simulink model "branch_offset_rate210_20161217_000202"  (R2014a)
settings: Solver=FixedStepDiscrete  SolverMode=SingleTasking  StartTime=0.0  StopTime=10.0  FixedStep=0.002  RelTol=1e-3
settings Model: BufferReuse=off  Creator=yoshi12  LastModifiedBy=yoshi12
settings OptimizationCC: BlockReduction=off  OptimizeBlockIOStorage=off  BufferReuse=off  GlobalBufferReuse=off  ExpressionFolding=off  LocalBlockOutputs=off  OptimizeModelRefInitCode=on  LifeSpan=1  SimCompilerOptimization=off
settings DebuggingCC: MergeDetectMultiDrivingBlocksExec=error  MultiTaskRateTransMsg=warning  FrameProcessingCompatibilityMsg=error
settings RTWCC: SystemTargetFile=ert.tlc  GenCodeOnly=on  TemplateMakefile=ert_default_tmf  Description=Embedded Coder  GenerateReport=on  IncludeHyperlinkInReport=on  LaunchReport=on  GenerateTraceInfo=on  GenerateTraceReport=on  GenerateTraceReportSl=on  GenerateTraceReportSf=on  GenerateTraceReportEml=on  RTWCompilerOptimization=off
settings CodeAppCC: IgnoreCustomStorageClasses=off
settings ERTTargetCC: ParMdlRefBuildCompliant=on  CompOptLevelCompliant=on  ConcurrentExecutionCompliant=on  ERTFirstTimeCompliant=on  ModelStepFunctionPrototypeControlCompliant=on  CPPClassGenCompliant=on  InlinedParameterPlacement=Hierarchical  ERTCustomFileTemplate=example_file_process.tlc
settings ConfigComp: CovMetricSettings=dw  CovHtmlReporting=on  CovSaveCumulativeToWorkspaceVar=on  CovSaveSingleToWorkspaceVar=on  CovModelRefEnable=Off  CovExternalEMLEnable=off  CovSFcnEnable=off

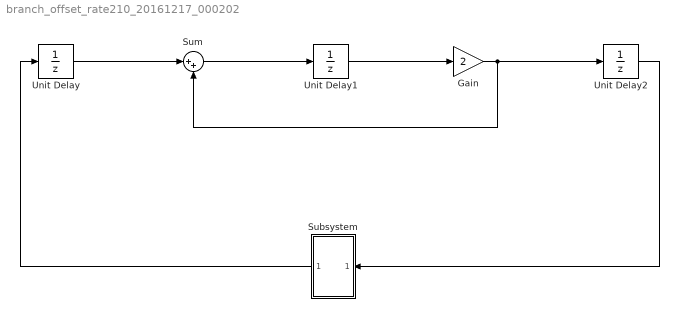
== system branch_offset_rate210_20161217_000202 ==
  Gain : Gain  Gain=2  SampleTime=0.002
  Subsystem : Subsystem
  Sum : Sum  Inputs=|++  SampleTime=0.002
  Unit Delay : UnitDelay  InitialCondition=1  SampleTime=-1
  Unit Delay1 : UnitDelay  InitialCondition=2  SampleTime=-1
  Unit Delay2 : UnitDelay  InitialCondition=1  SampleTime=-1
  wires:
  Unit Delay/1 -> Sum/1
  Sum/1 -> Unit Delay1/1
  Unit Delay1/1 -> Gain/1
  Gain/1 -> Sum/2, Unit Delay2/1
  Unit Delay2/1 -> Subsystem/1(In1)
  Subsystem/1(Out1) -> Unit Delay/1

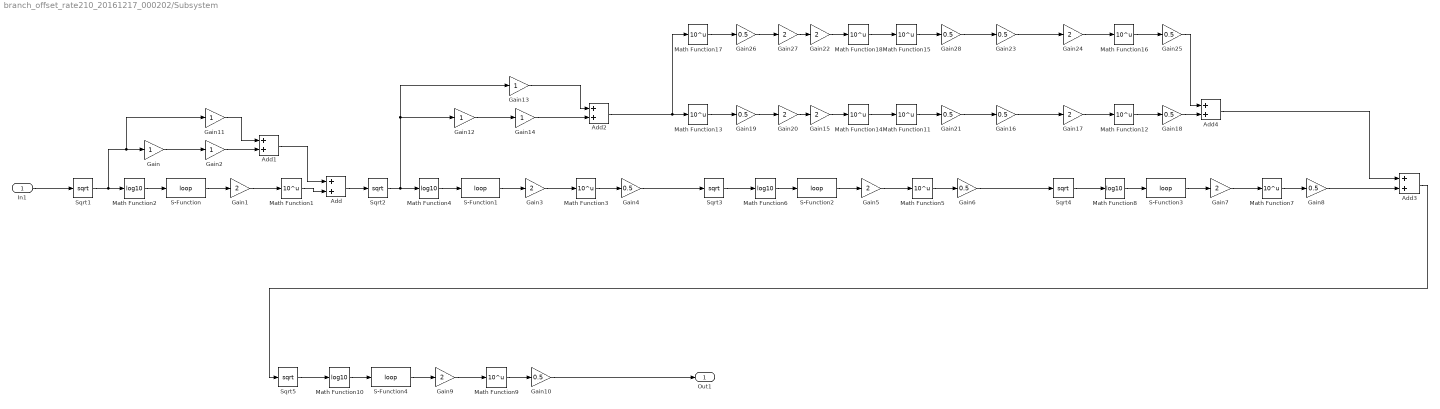
== system branch_offset_rate210_20161217_000202/Subsystem ==
  In1 : Inport
  Add{,1..2,4} (4 alike) : Sum  SampleTime=[0.01,0]
  Add3 : Sum  SampleTime=[0.01,0.006]
  Gain{,2,11..14} (6 alike) : Gain  SampleTime=[0.01,0]
  Gain1 : Gain  Gain=2  SampleTime=[0.01,0]
  Gain10 : Gain  Gain=0.5  SampleTime=[0.01,0.008]
  Gain{7,15,17,20,22,24,27} (7 alike) : Gain  Gain=2  SampleTime=[0.01,0.006]
  Gain{8,16,18..19,21,23,25..26,28} (9 alike) : Gain  Gain=0.5  SampleTime=[0.01,0.006]
  Gain3 : Gain  Gain=2  SampleTime=[0.01,0.002]
  Gain4 : Gain  Gain=0.5  SampleTime=[0.01,0.002]
  Gain5 : Gain  Gain=2  SampleTime=[0.01,0.004]
  Gain6 : Gain  Gain=0.5  SampleTime=[0.01,0.004]
  Gain9 : Gain  Gain=2  SampleTime=[0.01,0.008]
  Math Function1 : Math  Operator=10^u  SampleTime=[0.01,0]  SaturateOnIntegerOverflow=on
  Math Function10 : Math  Operator=log10  SampleTime=[0.01,0.008]  SaturateOnIntegerOverflow=on
  Math Function{7,11..18} (9 alike) : Math  Operator=10^u  SampleTime=[0.01,0.006]  SaturateOnIntegerOverflow=on
  Math Function2 : Math  Operator=log10  SampleTime=[0.01,0]  SaturateOnIntegerOverflow=on
  Math Function3 : Math  Operator=10^u  SampleTime=[0.01,0.002]  SaturateOnIntegerOverflow=on
  Math Function4 : Math  Operator=log10  SampleTime=[0.01,0.002]  SaturateOnIntegerOverflow=on
  Math Function5 : Math  Operator=10^u  SampleTime=[0.01,0.004]  SaturateOnIntegerOverflow=on
  Math Function6 : Math  Operator=log10  SampleTime=[0.01,0.004]  SaturateOnIntegerOverflow=on
  Math Function8 : Math  Operator=log10  SampleTime=[0.01,0.006]  SaturateOnIntegerOverflow=on
  Math Function9 : Math  Operator=10^u  SampleTime=[0.01,0.008]  SaturateOnIntegerOverflow=on
  S-Function{,1..4} (5 alike) : S-Function  FunctionName=loop  EnableBusSupport=off
  Sqrt1 : Sqrt  SampleTime=[0.01,0]  SaturateOnIntegerOverflow=on
  Sqrt2 : Sqrt  SampleTime=[0.01,0.002]  SaturateOnIntegerOverflow=on
  Sqrt3 : Sqrt  SampleTime=[0.01,0.004]  SaturateOnIntegerOverflow=on
  Sqrt4 : Sqrt  SampleTime=[0.01,0.006]  SaturateOnIntegerOverflow=on
  Sqrt5 : Sqrt  SampleTime=[0.01,0.008]  SaturateOnIntegerOverflow=on
  Out1 : Outport
  wires:
  Math Function3/1 -> Gain4/1
  Math Function8/1 -> S-Function3/1
  Sqrt1/1 -> Gain11/1, Gain/1, Math Function2/1
  Math Function10/1 -> S-Function4/1
  Gain9/1 -> Math Function9/1
  Math Function1/1 -> Add/2
  S-Function2/1 -> Gain5/1
  Math Function9/1 -> Gain10/1
  Gain10/1 -> Out1/1
  Sqrt3/1 -> Math Function6/1
  Sqrt4/1 -> Math Function8/1
  Gain3/1 -> Math Function3/1
  Gain6/1 -> Sqrt4/1
  Math Function5/1 -> Gain6/1
  Add/1 -> Sqrt2/1
  Math Function4/1 -> S-Function1/1
  Gain1/1 -> Math Function1/1
  Math Function2/1 -> S-Function/1
  S-Function3/1 -> Gain7/1
  Gain5/1 -> Math Function5/1
  Sqrt2/1 -> Math Function4/1, Gain13/1, Gain12/1
  S-Function4/1 -> Gain9/1
  S-Function/1 -> Gain1/1
  Sqrt5/1 -> Math Function10/1
  Math Function7/1 -> Gain8/1
  Gain7/1 -> Math Function7/1
  Math Function6/1 -> S-Function2/1
  Add3/1 -> Sqrt5/1
  S-Function1/1 -> Gain3/1
  In1/1 -> Sqrt1/1
  Gain4/1 -> Sqrt3/1
  Gain/1 -> Gain2/1
  Gain2/1 -> Add1/2
  Gain11/1 -> Add1/1
  Add1/1 -> Add/1
  Gain12/1 -> Gain14/1
  Gain14/1 -> Add2/2
  Gain13/1 -> Add2/1
  Add2/1 -> Math Function17/1, Math Function13/1
  Gain8/1 -> Add3/2
  Gain21/1 -> Gain16/1
  Gain16/1 -> Gain17/1
  Gain17/1 -> Math Function12/1
  Gain18/1 -> Add4/2
  Math Function12/1 -> Gain18/1
  Gain19/1 -> Gain20/1
  Math Function13/1 -> Gain19/1
  Gain20/1 -> Gain15/1
  Gain15/1 -> Math Function14/1
  Math Function14/1 -> Math Function11/1
  Math Function11/1 -> Gain21/1
  Add4/1 -> Add3/1
  Gain28/1 -> Gain23/1
  Gain23/1 -> Gain24/1
  Gain24/1 -> Math Function16/1
  Math Function16/1 -> Gain25/1
  Gain26/1 -> Gain27/1
  Math Function17/1 -> Gain26/1
  Gain27/1 -> Gain22/1
  Gain22/1 -> Math Function18/1
  Math Function18/1 -> Math Function15/1
  Math Function15/1 -> Gain28/1
  Gain25/1 -> Add4/1
